simulink model "gait_testing"  (R2024a)
settings: Solver=ode23t  StartTime=0.0  StopTime=8  RelTol=1e-3  AbsTol=1e-3  EnableMultiTasking=on
model workspace (MAT data in the model file):
  A = 0.4
  Length_torso : Simulink.Parameter (value not decoded)
  Lower_limbs : Simulink.Parameter (value not decoded)
  Upper_limbs : Simulink.Parameter (value not decoded)
  Width_torso : Simulink.Parameter (value not decoded)
  f = 1.5
  r_foot : Simulink.Parameter (value not decoded)
  t_leg : Simulink.Parameter (value not decoded)
symbols that are objects in the model workspace (value not decoded): Length_torso, Lower_limbs, t_leg, Upper_limbs, Width_torso
undefined symbols (not defined in the file): P0x, P0z, P1x, P1z, P2x, P2z, X, Y, Z
libraries: sm_lib x88, functionAngles x16, functionAnglesSide x16, nesl_utility x15
(part 8 of 10)

== system gait_testing/Gait Selector/Trot Gait - Drive Function/left Front Hip gait/If Action Subsystem1 ==
  In1 : Inport
  tdur : Inport  Port=2
  Add : Sum  Inputs=+-
  Constant : Constant  Value=1.0 * pi
  Divide : Product  Inputs=*/
  Gain1 : Gain  Gain=2
  Gain4 : Gain  Gain=2*pi
  Sin : Trigonometry
  Out1 : Outport
  wires:
  Sin/1 -> Out1/1
  In1/1 -> Gain4/1
  Add/1 -> Gain1/1
  Constant/1 -> Add/2
  Gain1/1 -> Sin/1
  Gain4/1 -> Divide/1
  Divide/1 -> Add/1
  tdur/1 -> Divide/2

== system gait_testing/Gait Selector/Trot Gait - Drive Function/left Front Hip gait/If Action Subsystem2 ==
  In1 : Inport
  tdur : Inport  Port=2
  Add : Sum  Inputs=+-
  Constant : Constant  Value=1.25 * pi
  Divide : Product  Inputs=*/
  Gain1 : Gain  Gain=2/3
  Gain4 : Gain  Gain=2*pi
  Sin : Trigonometry  Operator=cos
  Out1 : Outport
  wires:
  Sin/1 -> Out1/1
  In1/1 -> Gain4/1
  Add/1 -> Gain1/1
  Constant/1 -> Add/2
  Gain1/1 -> Sin/1
  Gain4/1 -> Divide/1
  Divide/1 -> Add/1
  tdur/1 -> Divide/2

== system gait_testing/Gait Selector/Trot Gait - Drive Function/left Front Knee gait/If Action Subsystem4 ==
  In1 : Inport
  tdur : Inport  Port=2
  Add : Sum  Inputs=+-
  Constant : Constant  Value=0.75 * pi
  Divide : Product  Inputs=*/
  Gain1 : Gain  Gain=2
  Gain4 : Gain  Gain=2*pi
  Sin : Trigonometry
  Out1 : Outport
  wires:
  Sin/1 -> Out1/1
  In1/1 -> Gain4/1
  Add/1 -> Gain1/1
  Constant/1 -> Add/2
  Gain1/1 -> Sin/1
  Divide/1 -> Add/1
  Gain4/1 -> Divide/1
  tdur/1 -> Divide/2

== system gait_testing/Gait Selector/Trot Gait - Drive Function/right Back Hip gait/If Action Subsystem ==
  In1 : Inport
  tdur : Inport  Port=2
  Add : Sum  Inputs=+-
  Constant : Constant  Value=1.5 * pi
  Divide : Product  Inputs=*/
  Gain1 : Gain  Gain=2/3
  Gain4 : Gain  Gain=2*pi
  Sin : Trigonometry
  Out1 : Outport
  wires:
  In1/1 -> Gain4/1
  Constant/1 -> Add/2
  Add/1 -> Gain1/1
  Gain1/1 -> Sin/1
  Sin/1 -> Out1/1
  Gain4/1 -> Divide/1
  tdur/1 -> Divide/2
  Divide/1 -> Add/1

== system gait_testing/Gait Selector/Trot Gait - Drive Function/right Back Hip gait/If Action Subsystem1 ==
  In1 : Inport
  tdur : Inport  Port=2
  Add : Sum  Inputs=+-
  Constant : Constant  Value=1.0 * pi
  Divide : Product  Inputs=*/
  Gain1 : Gain  Gain=2
  Gain4 : Gain  Gain=2*pi
  Sin : Trigonometry
  Out1 : Outport
  wires:
  Sin/1 -> Out1/1
  In1/1 -> Gain4/1
  Add/1 -> Gain1/1
  Constant/1 -> Add/2
  Gain1/1 -> Sin/1
  Gain4/1 -> Divide/1
  Divide/1 -> Add/1
  tdur/1 -> Divide/2

== system gait_testing/Gait Selector/Trot Gait - Drive Function/right Back Hip gait/If Action Subsystem2 ==
  In1 : Inport
  tdur : Inport  Port=2
  Add : Sum  Inputs=+-
  Constant : Constant  Value=1.25 * pi
  Divide : Product  Inputs=*/
  Gain1 : Gain  Gain=2/3
  Gain4 : Gain  Gain=2*pi
  Sin : Trigonometry  Operator=cos
  Out1 : Outport
  wires:
  Sin/1 -> Out1/1
  In1/1 -> Gain4/1
  Add/1 -> Gain1/1
  Constant/1 -> Add/2
  Gain1/1 -> Sin/1
  Gain4/1 -> Divide/1
  Divide/1 -> Add/1
  tdur/1 -> Divide/2

== system gait_testing/Gait Selector/Trot Gait - Drive Function/right Back Knee gait/If Action Subsystem4 ==
  In1 : Inport
  tdur : Inport  Port=2
  Add : Sum  Inputs=+-
  Constant : Constant  Value=0.75 * pi
  Divide : Product  Inputs=*/
  Gain1 : Gain  Gain=2
  Gain4 : Gain  Gain=2*pi
  Sin : Trigonometry
  Out1 : Outport
  wires:
  Sin/1 -> Out1/1
  In1/1 -> Gain4/1
  Add/1 -> Gain1/1
  Constant/1 -> Add/2
  Gain1/1 -> Sin/1
  Divide/1 -> Add/1
  Gain4/1 -> Divide/1
  tdur/1 -> Divide/2

== system gait_testing/Gait Selector/Trot Gait - Drive Function/right Front Hip gait/If Action Subsystem ==
  In1 : Inport
  tdur : Inport  Port=2
  Add : Sum  Inputs=+-
  Constant : Constant  Value=1.5 * pi
  Divide : Product  Inputs=*/
  Gain1 : Gain  Gain=2/3
  Gain4 : Gain  Gain=2*pi
  Sin : Trigonometry
  Out1 : Outport
  wires:
  In1/1 -> Gain4/1
  Constant/1 -> Add/2
  Add/1 -> Gain1/1
  Gain1/1 -> Sin/1
  Sin/1 -> Out1/1
  Gain4/1 -> Divide/1
  tdur/1 -> Divide/2
  Divide/1 -> Add/1

== system gait_testing/Gait Selector/Trot Gait - Drive Function/right Front Hip gait/If Action Subsystem1 ==
  In1 : Inport
  tdur : Inport  Port=2
  Add : Sum  Inputs=+-
  Constant : Constant  Value=1.0 * pi
  Divide : Product  Inputs=*/
  Gain1 : Gain  Gain=2
  Gain4 : Gain  Gain=2*pi
  Sin : Trigonometry
  Out1 : Outport
  wires:
  Sin/1 -> Out1/1
  In1/1 -> Gain4/1
  Add/1 -> Gain1/1
  Constant/1 -> Add/2
  Gain1/1 -> Sin/1
  Gain4/1 -> Divide/1
  Divide/1 -> Add/1
  tdur/1 -> Divide/2

== system gait_testing/Gait Selector/Trot Gait - Drive Function/right Front Hip gait/If Action Subsystem2 ==
  In1 : Inport
  tdur : Inport  Port=2
  Add : Sum  Inputs=+-
  Constant : Constant  Value=1.25 * pi
  Divide : Product  Inputs=*/
  Gain1 : Gain  Gain=2/3
  Gain4 : Gain  Gain=2*pi
  Sin : Trigonometry  Operator=cos
  Out1 : Outport
  wires:
  Sin/1 -> Out1/1
  In1/1 -> Gain4/1
  Add/1 -> Gain1/1
  Constant/1 -> Add/2
  Gain1/1 -> Sin/1
  Gain4/1 -> Divide/1
  Divide/1 -> Add/1
  tdur/1 -> Divide/2

== system gait_testing/Gait Selector/Trot Gait - Drive Function/right Front Knee gait/If Action Subsystem4 ==
  In1 : Inport
  tdur : Inport  Port=2
  Add : Sum  Inputs=+-
  Constant : Constant  Value=0.75 * pi
  Divide : Product  Inputs=*/
  Gain1 : Gain  Gain=2
  Gain4 : Gain  Gain=2*pi
  Sin : Trigonometry
  Out1 : Outport
  wires:
  Sin/1 -> Out1/1
  In1/1 -> Gain4/1
  Add/1 -> Gain1/1
  Constant/1 -> Add/2
  Gain1/1 -> Sin/1
  Divide/1 -> Add/1
  Gain4/1 -> Divide/1
  tdur/1 -> Divide/2

== system gait_testing/Gait Selector/Turn Left Gait - Bezier Curves/Plane Movement/Subsystem1 ==
  X(t) : Inport
  Y(t) : Inport  Port=2
  Add : Sum  Inputs=+--+
  Add1 : Sum
  Add2 : Sum
  Asin : Trigonometry  Operator=asin
  Asin1 : Trigonometry  Operator=asin
  Cos : Trigonometry  Operator=acos
  Divide : Product  Inputs=*/
  Divide1 : Product  Inputs=*/
  Gain : Gain  Gain=1/(2*Upper_limbs*Lower_limbs)
  Gain1 : Gain  Gain=Lower_limbs
  Length lower Limb : Constant  Value=Lower_limbs
  Length upper Limb : Constant  Value=Upper_limbs
  Sin : Trigonometry
  Square{,1..3} (4 alike) : Math  Operator=square
  Square Root : Sqrt
  Theta1(X,Y) : Outport
  Theta2(X,Y) : Outport  Port=2
  wires:
  X(t)/1 -> Divide/1, Square/1
  Y(t)/1 -> Square1/1
  Square/1 -> Add1/1, Add/1
  Length upper Limb/1 -> Square2/1
  Length lower Limb/1 -> Square3/1
  Square2/1 -> Add/2
  Square3/1 -> Add/3
  Square1/1 -> Add1/2, Add/4
  Add/1 -> Gain/1
  Gain/1 -> Cos/1
  Cos/1 -> Theta2(X,Y)/1, Sin/1
  Asin/1 -> Add2/1
  Sin/1 -> Gain1/1
  Add1/1 -> Square Root/1
  Gain1/1 -> Divide1/1
  Square Root/1 -> Divide/2, Divide1/2
  Divide1/1 -> Asin1/1
  Asin1/1 -> Add2/2
  Add2/1 -> Theta1(X,Y)/1
  Divide/1 -> Asin/1

== system gait_testing/Gait Selector/Turn Left Gait - Bezier Curves/Plane Movement1/Subsystem1 ==
  X(t) : Inport
  Y(t) : Inport  Port=2
  Add : Sum  Inputs=+--+
  Add1 : Sum
  Add2 : Sum
  Asin : Trigonometry  Operator=asin
  Asin1 : Trigonometry  Operator=asin
  Cos : Trigonometry  Operator=acos
  Divide : Product  Inputs=*/
  Divide1 : Product  Inputs=*/
  Gain : Gain  Gain=1/(2*Upper_limbs*Lower_limbs)
  Gain1 : Gain  Gain=Lower_limbs
  Length lower Limb : Constant  Value=Lower_limbs
  Length upper Limb : Constant  Value=Upper_limbs
  Sin : Trigonometry
  Square{,1..3} (4 alike) : Math  Operator=square
  Square Root : Sqrt
  Theta1(X,Y) : Outport
  Theta2(X,Y) : Outport  Port=2
  wires:
  X(t)/1 -> Divide/1, Square/1
  Y(t)/1 -> Square1/1
  Square/1 -> Add1/1, Add/1
  Length upper Limb/1 -> Square2/1
  Length lower Limb/1 -> Square3/1
  Square2/1 -> Add/2
  Square3/1 -> Add/3
  Square1/1 -> Add1/2, Add/4
  Add/1 -> Gain/1
  Gain/1 -> Cos/1
  Cos/1 -> Theta2(X,Y)/1, Sin/1
  Asin/1 -> Add2/1
  Sin/1 -> Gain1/1
  Add1/1 -> Square Root/1
  Gain1/1 -> Divide1/1
  Square Root/1 -> Divide/2, Divide1/2
  Divide1/1 -> Asin1/1
  Asin1/1 -> Add2/2
  Add2/1 -> Theta1(X,Y)/1
  Divide/1 -> Asin/1

== system gait_testing/Gait Selector/Turn Left Gait - Bezier Curves/Plane Movement2/Subsystem1 ==
  X(t) : Inport
  Y(t) : Inport  Port=2
  Add : Sum  Inputs=+--+
  Add1 : Sum
  Add2 : Sum
  Asin : Trigonometry  Operator=asin
  Asin1 : Trigonometry  Operator=asin
  Cos : Trigonometry  Operator=acos
  Divide : Product  Inputs=*/
  Divide1 : Product  Inputs=*/
  Gain : Gain  Gain=1/(2*Upper_limbs*Lower_limbs)
  Gain1 : Gain  Gain=Lower_limbs
  Length lower Limb : Constant  Value=Lower_limbs
  Length upper Limb : Constant  Value=Upper_limbs
  Sin : Trigonometry
  Square{,1..3} (4 alike) : Math  Operator=square
  Square Root : Sqrt
  Theta1(X,Y) : Outport
  Theta2(X,Y) : Outport  Port=2
  wires:
  Divide/1 -> Asin/1
  Add2/1 -> Theta1(X,Y)/1
  Asin1/1 -> Add2/2
  Divide1/1 -> Asin1/1
  Square Root/1 -> Divide1/2, Divide/2
  Gain1/1 -> Divide1/1
  Add1/1 -> Square Root/1
  Sin/1 -> Gain1/1
  Asin/1 -> Add2/1
  Cos/1 -> Sin/1, Theta2(X,Y)/1
  Gain/1 -> Cos/1
  Add/1 -> Gain/1
  Square1/1 -> Add/4, Add1/2
  Square3/1 -> Add/3
  Square2/1 -> Add/2
  Length lower Limb/1 -> Square3/1
  Length upper Limb/1 -> Square2/1
  Square/1 -> Add/1, Add1/1
  Y(t)/1 -> Square1/1
  X(t)/1 -> Square/1, Divide/1

== system gait_testing/Gait Selector/Turn Left Gait - Bezier Curves/Plane Movement3/Subsystem1 ==
  X(t) : Inport
  Y(t) : Inport  Port=2
  Add : Sum  Inputs=+--+
  Add1 : Sum
  Add2 : Sum
  Asin : Trigonometry  Operator=asin
  Asin1 : Trigonometry  Operator=asin
  Cos : Trigonometry  Operator=acos
  Divide : Product  Inputs=*/
  Divide1 : Product  Inputs=*/
  Gain : Gain  Gain=1/(2*Upper_limbs*Lower_limbs)
  Gain1 : Gain  Gain=Lower_limbs
  Length lower Limb : Constant  Value=Lower_limbs
  Length upper Limb : Constant  Value=Upper_limbs
  Sin : Trigonometry
  Square{,1..3} (4 alike) : Math  Operator=square
  Square Root : Sqrt
  Theta1(X,Y) : Outport
  Theta2(X,Y) : Outport  Port=2
  wires:
  X(t)/1 -> Divide/1, Square/1
  Y(t)/1 -> Square1/1
  Square/1 -> Add1/1, Add/1
  Length upper Limb/1 -> Square2/1
  Length lower Limb/1 -> Square3/1
  Square2/1 -> Add/2
  Square3/1 -> Add/3
  Square1/1 -> Add1/2, Add/4
  Add/1 -> Gain/1
  Gain/1 -> Cos/1
  Cos/1 -> Theta2(X,Y)/1, Sin/1
  Asin/1 -> Add2/1
  Sin/1 -> Gain1/1
  Add1/1 -> Square Root/1
  Gain1/1 -> Divide1/1
  Square Root/1 -> Divide/2, Divide1/2
  Divide1/1 -> Asin1/1
  Asin1/1 -> Add2/2
  Add2/1 -> Theta1(X,Y)/1
  Divide/1 -> Asin/1

== system gait_testing/Gait Selector/Turn Left Gait - Bezier Curves/Plane Movement4/Subsystem1 ==
  X(t) : Inport
  Y(t) : Inport  Port=2
  Add : Sum  Inputs=+--+
  Add1 : Sum
  Add2 : Sum
  Asin : Trigonometry  Operator=asin
  Asin1 : Trigonometry  Operator=asin
  Cos : Trigonometry  Operator=acos
  Divide : Product  Inputs=*/
  Divide1 : Product  Inputs=*/
  Gain : Gain  Gain=1/(2*Upper_limbs*Lower_limbs)
  Gain1 : Gain  Gain=Lower_limbs
  Length lower Limb : Constant  Value=Lower_limbs
  Length upper Limb : Constant  Value=Upper_limbs
  Sin : Trigonometry
  Square{,1..3} (4 alike) : Math  Operator=square
  Square Root : Sqrt
  Theta1(X,Y) : Outport
  Theta2(X,Y) : Outport  Port=2
  wires:
  Divide/1 -> Asin/1
  Add2/1 -> Theta1(X,Y)/1
  Asin1/1 -> Add2/2
  Divide1/1 -> Asin1/1
  Square Root/1 -> Divide1/2, Divide/2
  Gain1/1 -> Divide1/1
  Add1/1 -> Square Root/1
  Sin/1 -> Gain1/1
  Asin/1 -> Add2/1
  Cos/1 -> Sin/1, Theta2(X,Y)/1
  Gain/1 -> Cos/1
  Add/1 -> Gain/1
  Square1/1 -> Add/4, Add1/2
  Square3/1 -> Add/3
  Square2/1 -> Add/2
  Length lower Limb/1 -> Square3/1
  Length upper Limb/1 -> Square2/1
  Square/1 -> Add/1, Add1/1
  Y(t)/1 -> Square1/1
  X(t)/1 -> Square/1, Divide/1

== system gait_testing/Gait Selector/Turn Left Gait - Bezier Curves/Sin-Movement/Subsystem1 ==
  X(t) : Inport
  Y(t) : Inport  Port=2
  Add : Sum  Inputs=+--+
  Add1 : Sum
  Add2 : Sum
  Asin : Trigonometry  Operator=asin
  Asin1 : Trigonometry  Operator=asin
  Cos : Trigonometry  Operator=acos
  Divide : Product  Inputs=*/
  Divide1 : Product  Inputs=*/
  Gain : Gain  Gain=1/(2*Upper_limbs*Lower_limbs)
  Gain1 : Gain  Gain=Lower_limbs
  Length lower Limb : Constant  Value=Lower_limbs
  Length upper Limb : Constant  Value=Upper_limbs
  Sin : Trigonometry
  Square{,1..3} (4 alike) : Math  Operator=square
  Square Root : Sqrt
  Theta1(X,Y) : Outport
  Theta2(X,Y) : Outport  Port=2
  wires:
  X(t)/1 -> Divide/1, Square/1
  Y(t)/1 -> Square1/1
  Square/1 -> Add1/1, Add/1
  Length upper Limb/1 -> Square2/1
  Length lower Limb/1 -> Square3/1
  Square2/1 -> Add/2
  Square3/1 -> Add/3
  Square1/1 -> Add1/2, Add/4
  Add/1 -> Gain/1
  Gain/1 -> Cos/1
  Cos/1 -> Theta2(X,Y)/1, Sin/1
  Asin/1 -> Add2/1
  Sin/1 -> Gain1/1
  Add1/1 -> Square Root/1
  Gain1/1 -> Divide1/1
  Square Root/1 -> Divide/2, Divide1/2
  Divide1/1 -> Asin1/1
  Asin1/1 -> Add2/2
  Add2/1 -> Theta1(X,Y)/1
  Divide/1 -> Asin/1

== system gait_testing/Gait Selector/Turn Left Gait - Bezier Curves/Stop when change/Triggered Subsystem ==
  t : Inport
  Action Port : ActionPort  InitializeStates=reset  ActionPortLabel=case [ 1 ]:
  MATLAB Function : MATLAB Function  TreatAsAtomicUnit=on
  Change Time : Outport
  wires:
  MATLAB Function/1(activationTime) -> Change Time/1
  t/1 -> MATLAB Function/1(u)

== system gait_testing/Gait Selector/Turn Left Gait - Bezier Curves/delay and stop when change/Triggered Subsystem ==
  t : Inport
  Action Port : ActionPort  InitializeStates=reset  ActionPortLabel=case [ 1 ]:
  MATLAB Function : MATLAB Function  TreatAsAtomicUnit=on
  Change Time : Outport
  wires:
  MATLAB Function/1(activationTime) -> Change Time/1
  t/1 -> MATLAB Function/1(u)

== system gait_testing/Gait Selector/Turn Left Gait - Bezier Curves/delay and stop when change1/Triggered Subsystem ==
  t : Inport
  Action Port : ActionPort  InitializeStates=reset  ActionPortLabel=case [ 1 ]:
  MATLAB Function : MATLAB Function  TreatAsAtomicUnit=on
  Change Time : Outport
  wires:
  MATLAB Function/1(activationTime) -> Change Time/1
  t/1 -> MATLAB Function/1(u)

== system gait_testing/Gait Selector/Turn Left Gait - Bezier Curves/delay and stop when change2/Triggered Subsystem ==
  t : Inport
  Action Port : ActionPort  InitializeStates=reset  ActionPortLabel=case [ 1 ]:
  MATLAB Function : MATLAB Function  TreatAsAtomicUnit=on
  Change Time : Outport
  wires:
  MATLAB Function/1(activationTime) -> Change Time/1
  t/1 -> MATLAB Function/1(u)

== system gait_testing/Gait Selector/Turn Right Gait - Bezier Curves/Plane Movement/Subsystem1 ==
  X(t) : Inport
  Y(t) : Inport  Port=2
  Add : Sum  Inputs=+--+
  Add1 : Sum
  Add2 : Sum
  Asin : Trigonometry  Operator=asin
  Asin1 : Trigonometry  Operator=asin
  Cos : Trigonometry  Operator=acos
  Divide : Product  Inputs=*/
  Divide1 : Product  Inputs=*/
  Gain : Gain  Gain=1/(2*Upper_limbs*Lower_limbs)
  Gain1 : Gain  Gain=Lower_limbs
  Length lower Limb : Constant  Value=Lower_limbs
  Length upper Limb : Constant  Value=Upper_limbs
  Sin : Trigonometry
  Square{,1..3} (4 alike) : Math  Operator=square
  Square Root : Sqrt
  Theta1(X,Y) : Outport
  Theta2(X,Y) : Outport  Port=2
  wires:
  Divide/1 -> Asin/1
  Add2/1 -> Theta1(X,Y)/1
  Asin1/1 -> Add2/2
  Divide1/1 -> Asin1/1
  Square Root/1 -> Divide1/2, Divide/2
  Gain1/1 -> Divide1/1
  Add1/1 -> Square Root/1
  Sin/1 -> Gain1/1
  Asin/1 -> Add2/1
  Cos/1 -> Sin/1, Theta2(X,Y)/1
  Gain/1 -> Cos/1
  Add/1 -> Gain/1
  Square1/1 -> Add/4, Add1/2
  Square3/1 -> Add/3
  Square2/1 -> Add/2
  Length lower Limb/1 -> Square3/1
  Length upper Limb/1 -> Square2/1
  Square/1 -> Add/1, Add1/1
  Y(t)/1 -> Square1/1
  X(t)/1 -> Square/1, Divide/1

== system gait_testing/Gait Selector/Turn Right Gait - Bezier Curves/Plane Movement1/Subsystem1 ==
  X(t) : Inport
  Y(t) : Inport  Port=2
  Add : Sum  Inputs=+--+
  Add1 : Sum
  Add2 : Sum
  Asin : Trigonometry  Operator=asin
  Asin1 : Trigonometry  Operator=asin
  Cos : Trigonometry  Operator=acos
  Divide : Product  Inputs=*/
  Divide1 : Product  Inputs=*/
  Gain : Gain  Gain=1/(2*Upper_limbs*Lower_limbs)
  Gain1 : Gain  Gain=Lower_limbs
  Length lower Limb : Constant  Value=Lower_limbs
  Length upper Limb : Constant  Value=Upper_limbs
  Sin : Trigonometry
  Square{,1..3} (4 alike) : Math  Operator=square
  Square Root : Sqrt
  Theta1(X,Y) : Outport
  Theta2(X,Y) : Outport  Port=2
  wires:
  Divide/1 -> Asin/1
  Add2/1 -> Theta1(X,Y)/1
  Asin1/1 -> Add2/2
  Divide1/1 -> Asin1/1
  Square Root/1 -> Divide1/2, Divide/2
  Gain1/1 -> Divide1/1
  Add1/1 -> Square Root/1
  Sin/1 -> Gain1/1
  Asin/1 -> Add2/1
  Cos/1 -> Sin/1, Theta2(X,Y)/1
  Gain/1 -> Cos/1
  Add/1 -> Gain/1
  Square1/1 -> Add/4, Add1/2
  Square3/1 -> Add/3
  Square2/1 -> Add/2
  Length lower Limb/1 -> Square3/1
  Length upper Limb/1 -> Square2/1
  Square/1 -> Add/1, Add1/1
  Y(t)/1 -> Square1/1
  X(t)/1 -> Square/1, Divide/1

== system gait_testing/Gait Selector/Turn Right Gait - Bezier Curves/Plane Movement2/Subsystem1 ==
  X(t) : Inport
  Y(t) : Inport  Port=2
  Add : Sum  Inputs=+--+
  Add1 : Sum
  Add2 : Sum
  Asin : Trigonometry  Operator=asin
  Asin1 : Trigonometry  Operator=asin
  Cos : Trigonometry  Operator=acos
  Divide : Product  Inputs=*/
  Divide1 : Product  Inputs=*/
  Gain : Gain  Gain=1/(2*Upper_limbs*Lower_limbs)
  Gain1 : Gain  Gain=Lower_limbs
  Length lower Limb : Constant  Value=Lower_limbs
  Length upper Limb : Constant  Value=Upper_limbs
  Sin : Trigonometry
  Square{,1..3} (4 alike) : Math  Operator=square
  Square Root : Sqrt
  Theta1(X,Y) : Outport
  Theta2(X,Y) : Outport  Port=2
  wires:
  X(t)/1 -> Divide/1, Square/1
  Y(t)/1 -> Square1/1
  Square/1 -> Add1/1, Add/1
  Length upper Limb/1 -> Square2/1
  Length lower Limb/1 -> Square3/1
  Square2/1 -> Add/2
  Square3/1 -> Add/3
  Square1/1 -> Add1/2, Add/4
  Add/1 -> Gain/1
  Gain/1 -> Cos/1
  Cos/1 -> Theta2(X,Y)/1, Sin/1
  Asin/1 -> Add2/1
  Sin/1 -> Gain1/1
  Add1/1 -> Square Root/1
  Gain1/1 -> Divide1/1
  Square Root/1 -> Divide/2, Divide1/2
  Divide1/1 -> Asin1/1
  Asin1/1 -> Add2/2
  Add2/1 -> Theta1(X,Y)/1
  Divide/1 -> Asin/1

== system gait_testing/Gait Selector/Turn Right Gait - Bezier Curves/Plane Movement3/Subsystem1 ==
  X(t) : Inport
  Y(t) : Inport  Port=2
  Add : Sum  Inputs=+--+
  Add1 : Sum
  Add2 : Sum
  Asin : Trigonometry  Operator=asin
  Asin1 : Trigonometry  Operator=asin
  Cos : Trigonometry  Operator=acos
  Divide : Product  Inputs=*/
  Divide1 : Product  Inputs=*/
  Gain : Gain  Gain=1/(2*Upper_limbs*Lower_limbs)
  Gain1 : Gain  Gain=Lower_limbs
  Length lower Limb : Constant  Value=Lower_limbs
  Length upper Limb : Constant  Value=Upper_limbs
  Sin : Trigonometry
  Square{,1..3} (4 alike) : Math  Operator=square
  Square Root : Sqrt
  Theta1(X,Y) : Outport
  Theta2(X,Y) : Outport  Port=2
  wires:
  X(t)/1 -> Divide/1, Square/1
  Y(t)/1 -> Square1/1
  Square/1 -> Add1/1, Add/1
  Length upper Limb/1 -> Square2/1
  Length lower Limb/1 -> Square3/1
  Square2/1 -> Add/2
  Square3/1 -> Add/3
  Square1/1 -> Add1/2, Add/4
  Add/1 -> Gain/1
  Gain/1 -> Cos/1
  Cos/1 -> Theta2(X,Y)/1, Sin/1
  Asin/1 -> Add2/1
  Sin/1 -> Gain1/1
  Add1/1 -> Square Root/1
  Gain1/1 -> Divide1/1
  Square Root/1 -> Divide/2, Divide1/2
  Divide1/1 -> Asin1/1
  Asin1/1 -> Add2/2
  Add2/1 -> Theta1(X,Y)/1
  Divide/1 -> Asin/1

== system gait_testing/Gait Selector/Turn Right Gait - Bezier Curves/Plane Movement4/Subsystem1 ==
  X(t) : Inport
  Y(t) : Inport  Port=2
  Add : Sum  Inputs=+--+
  Add1 : Sum
  Add2 : Sum
  Asin : Trigonometry  Operator=asin
  Asin1 : Trigonometry  Operator=asin
  Cos : Trigonometry  Operator=acos
  Divide : Product  Inputs=*/
  Divide1 : Product  Inputs=*/
  Gain : Gain  Gain=1/(2*Upper_limbs*Lower_limbs)
  Gain1 : Gain  Gain=Lower_limbs
  Length lower Limb : Constant  Value=Lower_limbs
  Length upper Limb : Constant  Value=Upper_limbs
  Sin : Trigonometry
  Square{,1..3} (4 alike) : Math  Operator=square
  Square Root : Sqrt
  Theta1(X,Y) : Outport
  Theta2(X,Y) : Outport  Port=2
  wires:
  X(t)/1 -> Divide/1, Square/1
  Y(t)/1 -> Square1/1
  Square/1 -> Add1/1, Add/1
  Length upper Limb/1 -> Square2/1
  Length lower Limb/1 -> Square3/1
  Square2/1 -> Add/2
  Square3/1 -> Add/3
  Square1/1 -> Add1/2, Add/4
  Add/1 -> Gain/1
  Gain/1 -> Cos/1
  Cos/1 -> Theta2(X,Y)/1, Sin/1
  Asin/1 -> Add2/1
  Sin/1 -> Gain1/1
  Add1/1 -> Square Root/1
  Gain1/1 -> Divide1/1
  Square Root/1 -> Divide/2, Divide1/2
  Divide1/1 -> Asin1/1
  Asin1/1 -> Add2/2
  Add2/1 -> Theta1(X,Y)/1
  Divide/1 -> Asin/1

== system gait_testing/Gait Selector/Turn Right Gait - Bezier Curves/Sin-Movement/Subsystem1 ==
  X(t) : Inport
  Y(t) : Inport  Port=2
  Add : Sum  Inputs=+--+
  Add1 : Sum
  Add2 : Sum
  Asin : Trigonometry  Operator=asin
  Asin1 : Trigonometry  Operator=asin
  Cos : Trigonometry  Operator=acos
  Divide : Product  Inputs=*/
  Divide1 : Product  Inputs=*/
  Gain : Gain  Gain=1/(2*Upper_limbs*Lower_limbs)
  Gain1 : Gain  Gain=Lower_limbs
  Length lower Limb : Constant  Value=Lower_limbs
  Length upper Limb : Constant  Value=Upper_limbs
  Sin : Trigonometry
  Square{,1..3} (4 alike) : Math  Operator=square
  Square Root : Sqrt
  Theta1(X,Y) : Outport
  Theta2(X,Y) : Outport  Port=2
  wires:
  Divide/1 -> Asin/1
  Add2/1 -> Theta1(X,Y)/1
  Asin1/1 -> Add2/2
  Divide1/1 -> Asin1/1
  Square Root/1 -> Divide1/2, Divide/2
  Gain1/1 -> Divide1/1
  Add1/1 -> Square Root/1
  Sin/1 -> Gain1/1
  Asin/1 -> Add2/1
  Cos/1 -> Sin/1, Theta2(X,Y)/1
  Gain/1 -> Cos/1
  Add/1 -> Gain/1
  Square1/1 -> Add/4, Add1/2
  Square3/1 -> Add/3
  Square2/1 -> Add/2
  Length lower Limb/1 -> Square3/1
  Length upper Limb/1 -> Square2/1
  Square/1 -> Add/1, Add1/1
  Y(t)/1 -> Square1/1
  X(t)/1 -> Square/1, Divide/1

== system gait_testing/Gait Selector/Turn Right Gait - Bezier Curves/Stop when change/Triggered Subsystem ==
  t : Inport
  Action Port : ActionPort  InitializeStates=reset  ActionPortLabel=case [ 1 ]:
  MATLAB Function : MATLAB Function  TreatAsAtomicUnit=on
  Change Time : Outport
  wires:
  MATLAB Function/1(activationTime) -> Change Time/1
  t/1 -> MATLAB Function/1(u)

== system gait_testing/Gait Selector/Turn Right Gait - Bezier Curves/delay and stop when change/Triggered Subsystem ==
  t : Inport
  Action Port : ActionPort  InitializeStates=reset  ActionPortLabel=case [ 1 ]:
  MATLAB Function : MATLAB Function  TreatAsAtomicUnit=on
  Change Time : Outport
  wires:
  MATLAB Function/1(activationTime) -> Change Time/1
  t/1 -> MATLAB Function/1(u)

== system gait_testing/Gait Selector/Turn Right Gait - Bezier Curves/delay and stop when change1/Triggered Subsystem ==
  t : Inport
  Action Port : ActionPort  InitializeStates=reset  ActionPortLabel=case [ 1 ]:
  MATLAB Function : MATLAB Function  TreatAsAtomicUnit=on
  Change Time : Outport
  wires:
  MATLAB Function/1(activationTime) -> Change Time/1
  t/1 -> MATLAB Function/1(u)

== system gait_testing/Gait Selector/Turn Right Gait - Bezier Curves/delay and stop when change2/Triggered Subsystem ==
  t : Inport
  Action Port : ActionPort  InitializeStates=reset  ActionPortLabel=case [ 1 ]:
  MATLAB Function : MATLAB Function  TreatAsAtomicUnit=on
  Change Time : Outport
  wires:
  MATLAB Function/1(activationTime) -> Change Time/1
  t/1 -> MATLAB Function/1(u)

== system gait_testing/Gait Selector/Walk Back Gait - Bezier Curves/Plane Movement/Subsystem1 ==
  X(t) : Inport
  Y(t) : Inport  Port=2
  Add : Sum  Inputs=+--+
  Add1 : Sum
  Add2 : Sum
  Asin : Trigonometry  Operator=asin
  Asin1 : Trigonometry  Operator=asin
  Cos : Trigonometry  Operator=acos
  Divide : Product  Inputs=*/
  Divide1 : Product  Inputs=*/
  Gain : Gain  Gain=1/(2*Upper_limbs*Lower_limbs)
  Gain1 : Gain  Gain=Lower_limbs
  Length lower Limb : Constant  Value=Lower_limbs
  Length upper Limb : Constant  Value=Upper_limbs
  Sin : Trigonometry
  Square{,1..3} (4 alike) : Math  Operator=square
  Square Root : Sqrt
  Theta1(X,Y) : Outport
  Theta2(X,Y) : Outport  Port=2
  wires:
  Divide/1 -> Asin/1
  Add2/1 -> Theta1(X,Y)/1
  Asin1/1 -> Add2/2
  Divide1/1 -> Asin1/1
  Square Root/1 -> Divide1/2, Divide/2
  Gain1/1 -> Divide1/1
  Add1/1 -> Square Root/1
  Sin/1 -> Gain1/1
  Asin/1 -> Add2/1
  Cos/1 -> Sin/1, Theta2(X,Y)/1
  Gain/1 -> Cos/1
  Add/1 -> Gain/1
  Square1/1 -> Add/4, Add1/2
  Square3/1 -> Add/3
  Square2/1 -> Add/2
  Length lower Limb/1 -> Square3/1
  Length upper Limb/1 -> Square2/1
  Square/1 -> Add/1, Add1/1
  Y(t)/1 -> Square1/1
  X(t)/1 -> Square/1, Divide/1

== system gait_testing/Gait Selector/Walk Back Gait - Bezier Curves/Plane Movement1/Subsystem1 ==
  X(t) : Inport
  Y(t) : Inport  Port=2
  Add : Sum  Inputs=+--+
  Add1 : Sum
  Add2 : Sum
  Asin : Trigonometry  Operator=asin
  Asin1 : Trigonometry  Operator=asin
  Cos : Trigonometry  Operator=acos
  Divide : Product  Inputs=*/
  Divide1 : Product  Inputs=*/
  Gain : Gain  Gain=1/(2*Upper_limbs*Lower_limbs)
  Gain1 : Gain  Gain=Lower_limbs
  Length lower Limb : Constant  Value=Lower_limbs
  Length upper Limb : Constant  Value=Upper_limbs
  Sin : Trigonometry
  Square{,1..3} (4 alike) : Math  Operator=square
  Square Root : Sqrt
  Theta1(X,Y) : Outport
  Theta2(X,Y) : Outport  Port=2
  wires:
  Divide/1 -> Asin/1
  Add2/1 -> Theta1(X,Y)/1
  Asin1/1 -> Add2/2
  Divide1/1 -> Asin1/1
  Square Root/1 -> Divide1/2, Divide/2
  Gain1/1 -> Divide1/1
  Add1/1 -> Square Root/1
  Sin/1 -> Gain1/1
  Asin/1 -> Add2/1
  Cos/1 -> Sin/1, Theta2(X,Y)/1
  Gain/1 -> Cos/1
  Add/1 -> Gain/1
  Square1/1 -> Add/4, Add1/2
  Square3/1 -> Add/3
  Square2/1 -> Add/2
  Length lower Limb/1 -> Square3/1
  Length upper Limb/1 -> Square2/1
  Square/1 -> Add/1, Add1/1
  Y(t)/1 -> Square1/1
  X(t)/1 -> Square/1, Divide/1

== system gait_testing/Gait Selector/Walk Back Gait - Bezier Curves/Plane Movement2/Subsystem1 ==
  X(t) : Inport
  Y(t) : Inport  Port=2
  Add : Sum  Inputs=+--+
  Add1 : Sum
  Add2 : Sum
  Asin : Trigonometry  Operator=asin
  Asin1 : Trigonometry  Operator=asin
  Cos : Trigonometry  Operator=acos
  Divide : Product  Inputs=*/
  Divide1 : Product  Inputs=*/
  Gain : Gain  Gain=1/(2*Upper_limbs*Lower_limbs)
  Gain1 : Gain  Gain=Lower_limbs
  Length lower Limb : Constant  Value=Lower_limbs
  Length upper Limb : Constant  Value=Upper_limbs
  Sin : Trigonometry
  Square{,1..3} (4 alike) : Math  Operator=square
  Square Root : Sqrt
  Theta1(X,Y) : Outport
  Theta2(X,Y) : Outport  Port=2
  wires:
  X(t)/1 -> Divide/1, Square/1
  Y(t)/1 -> Square1/1
  Square/1 -> Add1/1, Add/1
  Length upper Limb/1 -> Square2/1
  Length lower Limb/1 -> Square3/1
  Square2/1 -> Add/2
  Square3/1 -> Add/3
  Square1/1 -> Add1/2, Add/4
  Add/1 -> Gain/1
  Gain/1 -> Cos/1
  Cos/1 -> Theta2(X,Y)/1, Sin/1
  Asin/1 -> Add2/1
  Sin/1 -> Gain1/1
  Add1/1 -> Square Root/1
  Gain1/1 -> Divide1/1
  Square Root/1 -> Divide/2, Divide1/2
  Divide1/1 -> Asin1/1
  Asin1/1 -> Add2/2
  Add2/1 -> Theta1(X,Y)/1
  Divide/1 -> Asin/1

== system gait_testing/Gait Selector/Walk Back Gait - Bezier Curves/Plane Movement3/Subsystem1 ==
  X(t) : Inport
  Y(t) : Inport  Port=2
  Add : Sum  Inputs=+--+
  Add1 : Sum
  Add2 : Sum
  Asin : Trigonometry  Operator=asin
  Asin1 : Trigonometry  Operator=asin
  Cos : Trigonometry  Operator=acos
  Divide : Product  Inputs=*/
  Divide1 : Product  Inputs=*/
  Gain : Gain  Gain=1/(2*Upper_limbs*Lower_limbs)
  Gain1 : Gain  Gain=Lower_limbs
  Length lower Limb : Constant  Value=Lower_limbs
  Length upper Limb : Constant  Value=Upper_limbs
  Sin : Trigonometry
  Square{,1..3} (4 alike) : Math  Operator=square
  Square Root : Sqrt
  Theta1(X,Y) : Outport
  Theta2(X,Y) : Outport  Port=2
  wires:
  Divide/1 -> Asin/1
  Add2/1 -> Theta1(X,Y)/1
  Asin1/1 -> Add2/2
  Divide1/1 -> Asin1/1
  Square Root/1 -> Divide1/2, Divide/2
  Gain1/1 -> Divide1/1
  Add1/1 -> Square Root/1
  Sin/1 -> Gain1/1
  Asin/1 -> Add2/1
  Cos/1 -> Sin/1, Theta2(X,Y)/1
  Gain/1 -> Cos/1
  Add/1 -> Gain/1
  Square1/1 -> Add/4, Add1/2
  Square3/1 -> Add/3
  Square2/1 -> Add/2
  Length lower Limb/1 -> Square3/1
  Length upper Limb/1 -> Square2/1
  Square/1 -> Add/1, Add1/1
  Y(t)/1 -> Square1/1
  X(t)/1 -> Square/1, Divide/1

== system gait_testing/Gait Selector/Walk Back Gait - Bezier Curves/Plane Movement4/Subsystem1 ==
  X(t) : Inport
  Y(t) : Inport  Port=2
  Add : Sum  Inputs=+--+
  Add1 : Sum
  Add2 : Sum
  Asin : Trigonometry  Operator=asin
  Asin1 : Trigonometry  Operator=asin
  Cos : Trigonometry  Operator=acos
  Divide : Product  Inputs=*/
  Divide1 : Product  Inputs=*/
  Gain : Gain  Gain=1/(2*Upper_limbs*Lower_limbs)
  Gain1 : Gain  Gain=Lower_limbs
  Length lower Limb : Constant  Value=Lower_limbs
  Length upper Limb : Constant  Value=Upper_limbs
  Sin : Trigonometry
  Square{,1..3} (4 alike) : Math  Operator=square
  Square Root : Sqrt
  Theta1(X,Y) : Outport
  Theta2(X,Y) : Outport  Port=2
  wires:
  X(t)/1 -> Divide/1, Square/1
  Y(t)/1 -> Square1/1
  Square/1 -> Add1/1, Add/1
  Length upper Limb/1 -> Square2/1
  Length lower Limb/1 -> Square3/1
  Square2/1 -> Add/2
  Square3/1 -> Add/3
  Square1/1 -> Add1/2, Add/4
  Add/1 -> Gain/1
  Gain/1 -> Cos/1
  Cos/1 -> Theta2(X,Y)/1, Sin/1
  Asin/1 -> Add2/1
  Sin/1 -> Gain1/1
  Add1/1 -> Square Root/1
  Gain1/1 -> Divide1/1
  Square Root/1 -> Divide/2, Divide1/2
  Divide1/1 -> Asin1/1
  Asin1/1 -> Add2/2
  Add2/1 -> Theta1(X,Y)/1
  Divide/1 -> Asin/1

== system gait_testing/Gait Selector/Walk Back Gait - Bezier Curves/Sin-Movement/Subsystem1 ==
  X(t) : Inport
  Y(t) : Inport  Port=2
  Add : Sum  Inputs=+--+
  Add1 : Sum
  Add2 : Sum
  Asin : Trigonometry  Operator=asin
  Asin1 : Trigonometry  Operator=asin
  Cos : Trigonometry  Operator=acos
  Divide : Product  Inputs=*/
  Divide1 : Product  Inputs=*/
  Gain : Gain  Gain=1/(2*Upper_limbs*Lower_limbs)
  Gain1 : Gain  Gain=Lower_limbs
  Length lower Limb : Constant  Value=Lower_limbs
  Length upper Limb : Constant  Value=Upper_limbs
  Sin : Trigonometry
  Square{,1..3} (4 alike) : Math  Operator=square
  Square Root : Sqrt
  Theta1(X,Y) : Outport
  Theta2(X,Y) : Outport  Port=2
  wires:
  Divide/1 -> Asin/1
  Add2/1 -> Theta1(X,Y)/1
  Asin1/1 -> Add2/2
  Divide1/1 -> Asin1/1
  Square Root/1 -> Divide1/2, Divide/2
  Gain1/1 -> Divide1/1
  Add1/1 -> Square Root/1
  Sin/1 -> Gain1/1
  Asin/1 -> Add2/1
  Cos/1 -> Sin/1, Theta2(X,Y)/1
  Gain/1 -> Cos/1
  Add/1 -> Gain/1
  Square1/1 -> Add/4, Add1/2
  Square3/1 -> Add/3
  Square2/1 -> Add/2
  Length lower Limb/1 -> Square3/1
  Length upper Limb/1 -> Square2/1
  Square/1 -> Add/1, Add1/1
  Y(t)/1 -> Square1/1
  X(t)/1 -> Square/1, Divide/1

== system gait_testing/Gait Selector/Walk Back Gait - Bezier Curves/Stop when change/Triggered Subsystem ==
  t : Inport
  Action Port : ActionPort  InitializeStates=reset  ActionPortLabel=case [ 1 ]:
  MATLAB Function : MATLAB Function  TreatAsAtomicUnit=on
  Change Time : Outport
  wires:
  MATLAB Function/1(activationTime) -> Change Time/1
  t/1 -> MATLAB Function/1(u)

== system gait_testing/Gait Selector/Walk Back Gait - Bezier Curves/delay and stop when change/Triggered Subsystem ==
  t : Inport
  Action Port : ActionPort  InitializeStates=reset  ActionPortLabel=case [ 1 ]:
  MATLAB Function : MATLAB Function  TreatAsAtomicUnit=on
  Change Time : Outport
  wires:
  MATLAB Function/1(activationTime) -> Change Time/1
  t/1 -> MATLAB Function/1(u)

== system gait_testing/Gait Selector/Walk Back Gait - Bezier Curves/delay and stop when change1/Triggered Subsystem ==
  t : Inport
  Action Port : ActionPort  InitializeStates=reset  ActionPortLabel=case [ 1 ]:
  MATLAB Function : MATLAB Function  TreatAsAtomicUnit=on
  Change Time : Outport
  wires:
  MATLAB Function/1(activationTime) -> Change Time/1
  t/1 -> MATLAB Function/1(u)

== system gait_testing/Gait Selector/Walk Back Gait - Bezier Curves/delay and stop when change2/Triggered Subsystem ==
  t : Inport
  Action Port : ActionPort  InitializeStates=reset  ActionPortLabel=case [ 1 ]:
  MATLAB Function : MATLAB Function  TreatAsAtomicUnit=on
  Change Time : Outport
  wires:
  MATLAB Function/1(activationTime) -> Change Time/1
  t/1 -> MATLAB Function/1(u)

== system gait_testing/Gait Selector/Walk Gait - Bezier Curves/Plane Movement/Subsystem1 ==
  X(t) : Inport
  Y(t) : Inport  Port=2
  Add : Sum  Inputs=+--+
  Add1 : Sum
  Add2 : Sum
  Asin : Trigonometry  Operator=asin
  Asin1 : Trigonometry  Operator=asin
  Cos : Trigonometry  Operator=acos
  Divide : Product  Inputs=*/
  Divide1 : Product  Inputs=*/
  Gain : Gain  Gain=1/(2*Upper_limbs*Lower_limbs)
  Gain1 : Gain  Gain=Lower_limbs
  Length lower Limb : Constant  Value=Lower_limbs
  Length upper Limb : Constant  Value=Upper_limbs
  Sin : Trigonometry
  Square{,1..3} (4 alike) : Math  Operator=square
  Square Root : Sqrt
  Theta1(X,Y) : Outport
  Theta2(X,Y) : Outport  Port=2
  wires:
  Divide/1 -> Asin/1
  Add2/1 -> Theta1(X,Y)/1
  Asin1/1 -> Add2/2
  Divide1/1 -> Asin1/1
  Square Root/1 -> Divide1/2, Divide/2
  Gain1/1 -> Divide1/1
  Add1/1 -> Square Root/1
  Sin/1 -> Gain1/1
  Asin/1 -> Add2/1
  Cos/1 -> Sin/1, Theta2(X,Y)/1
  Gain/1 -> Cos/1
  Add/1 -> Gain/1
  Square1/1 -> Add/4, Add1/2
  Square3/1 -> Add/3
  Square2/1 -> Add/2
  Length lower Limb/1 -> Square3/1
  Length upper Limb/1 -> Square2/1
  Square/1 -> Add/1, Add1/1
  Y(t)/1 -> Square1/1
  X(t)/1 -> Square/1, Divide/1

== system gait_testing/Gait Selector/Walk Gait - Bezier Curves/Plane Movement1/Subsystem1 ==
  X(t) : Inport
  Y(t) : Inport  Port=2
  Add : Sum  Inputs=+--+
  Add1 : Sum
  Add2 : Sum
  Asin : Trigonometry  Operator=asin
  Asin1 : Trigonometry  Operator=asin
  Cos : Trigonometry  Operator=acos
  Divide : Product  Inputs=*/
  Divide1 : Product  Inputs=*/
  Gain : Gain  Gain=1/(2*Upper_limbs*Lower_limbs)
  Gain1 : Gain  Gain=Lower_limbs
  Length lower Limb : Constant  Value=Lower_limbs
  Length upper Limb : Constant  Value=Upper_limbs
  Sin : Trigonometry
  Square{,1..3} (4 alike) : Math  Operator=square
  Square Root : Sqrt
  Theta1(X,Y) : Outport
  Theta2(X,Y) : Outport  Port=2
  wires:
  X(t)/1 -> Divide/1, Square/1
  Y(t)/1 -> Square1/1
  Square/1 -> Add1/1, Add/1
  Length upper Limb/1 -> Square2/1
  Length lower Limb/1 -> Square3/1
  Square2/1 -> Add/2
  Square3/1 -> Add/3
  Square1/1 -> Add1/2, Add/4
  Add/1 -> Gain/1
  Gain/1 -> Cos/1
  Cos/1 -> Theta2(X,Y)/1, Sin/1
  Asin/1 -> Add2/1
  Sin/1 -> Gain1/1
  Add1/1 -> Square Root/1
  Gain1/1 -> Divide1/1
  Square Root/1 -> Divide/2, Divide1/2
  Divide1/1 -> Asin1/1
  Asin1/1 -> Add2/2
  Add2/1 -> Theta1(X,Y)/1
  Divide/1 -> Asin/1

== system gait_testing/Gait Selector/Walk Gait - Bezier Curves/Plane Movement2/Subsystem1 ==
  X(t) : Inport
  Y(t) : Inport  Port=2
  Add : Sum  Inputs=+--+
  Add1 : Sum
  Add2 : Sum
  Asin : Trigonometry  Operator=asin
  Asin1 : Trigonometry  Operator=asin
  Cos : Trigonometry  Operator=acos
  Divide : Product  Inputs=*/
  Divide1 : Product  Inputs=*/
  Gain : Gain  Gain=1/(2*Upper_limbs*Lower_limbs)
  Gain1 : Gain  Gain=Lower_limbs
  Length lower Limb : Constant  Value=Lower_limbs
  Length upper Limb : Constant  Value=Upper_limbs
  Sin : Trigonometry
  Square{,1..3} (4 alike) : Math  Operator=square
  Square Root : Sqrt
  Theta1(X,Y) : Outport
  Theta2(X,Y) : Outport  Port=2
  wires:
  X(t)/1 -> Divide/1, Square/1
  Y(t)/1 -> Square1/1
  Square/1 -> Add1/1, Add/1
  Length upper Limb/1 -> Square2/1
  Length lower Limb/1 -> Square3/1
  Square2/1 -> Add/2
  Square3/1 -> Add/3
  Square1/1 -> Add1/2, Add/4
  Add/1 -> Gain/1
  Gain/1 -> Cos/1
  Cos/1 -> Theta2(X,Y)/1, Sin/1
  Asin/1 -> Add2/1
  Sin/1 -> Gain1/1
  Add1/1 -> Square Root/1
  Gain1/1 -> Divide1/1
  Square Root/1 -> Divide/2, Divide1/2
  Divide1/1 -> Asin1/1
  Asin1/1 -> Add2/2
  Add2/1 -> Theta1(X,Y)/1
  Divide/1 -> Asin/1

== system gait_testing/Gait Selector/Walk Gait - Bezier Curves/Plane Movement3/Subsystem1 ==
  X(t) : Inport
  Y(t) : Inport  Port=2
  Add : Sum  Inputs=+--+
  Add1 : Sum
  Add2 : Sum
  Asin : Trigonometry  Operator=asin
  Asin1 : Trigonometry  Operator=asin
  Cos : Trigonometry  Operator=acos
  Divide : Product  Inputs=*/
  Divide1 : Product  Inputs=*/
  Gain : Gain  Gain=1/(2*Upper_limbs*Lower_limbs)
  Gain1 : Gain  Gain=Lower_limbs
  Length lower Limb : Constant  Value=Lower_limbs
  Length upper Limb : Constant  Value=Upper_limbs
  Sin : Trigonometry
  Square{,1..3} (4 alike) : Math  Operator=square
  Square Root : Sqrt
  Theta1(X,Y) : Outport
  Theta2(X,Y) : Outport  Port=2
  wires:
  Divide/1 -> Asin/1
  Add2/1 -> Theta1(X,Y)/1
  Asin1/1 -> Add2/2
  Divide1/1 -> Asin1/1
  Square Root/1 -> Divide1/2, Divide/2
  Gain1/1 -> Divide1/1
  Add1/1 -> Square Root/1
  Sin/1 -> Gain1/1
  Asin/1 -> Add2/1
  Cos/1 -> Sin/1, Theta2(X,Y)/1
  Gain/1 -> Cos/1
  Add/1 -> Gain/1
  Square1/1 -> Add/4, Add1/2
  Square3/1 -> Add/3
  Square2/1 -> Add/2
  Length lower Limb/1 -> Square3/1
  Length upper Limb/1 -> Square2/1
  Square/1 -> Add/1, Add1/1
  Y(t)/1 -> Square1/1
  X(t)/1 -> Square/1, Divide/1

== system gait_testing/Gait Selector/Walk Gait - Bezier Curves/Plane Movement4/Subsystem1 ==
  X(t) : Inport
  Y(t) : Inport  Port=2
  Add : Sum  Inputs=+--+
  Add1 : Sum
  Add2 : Sum
  Asin : Trigonometry  Operator=asin
  Asin1 : Trigonometry  Operator=asin
  Cos : Trigonometry  Operator=acos
  Divide : Product  Inputs=*/
  Divide1 : Product  Inputs=*/
  Gain : Gain  Gain=1/(2*Upper_limbs*Lower_limbs)
  Gain1 : Gain  Gain=Lower_limbs
  Length lower Limb : Constant  Value=Lower_limbs
  Length upper Limb : Constant  Value=Upper_limbs
  Sin : Trigonometry
  Square{,1..3} (4 alike) : Math  Operator=square
  Square Root : Sqrt
  Theta1(X,Y) : Outport
  Theta2(X,Y) : Outport  Port=2
  wires:
  X(t)/1 -> Divide/1, Square/1
  Y(t)/1 -> Square1/1
  Square/1 -> Add1/1, Add/1
  Length upper Limb/1 -> Square2/1
  Length lower Limb/1 -> Square3/1
  Square2/1 -> Add/2
  Square3/1 -> Add/3
  Square1/1 -> Add1/2, Add/4
  Add/1 -> Gain/1
  Gain/1 -> Cos/1
  Cos/1 -> Theta2(X,Y)/1, Sin/1
  Asin/1 -> Add2/1
  Sin/1 -> Gain1/1
  Add1/1 -> Square Root/1
  Gain1/1 -> Divide1/1
  Square Root/1 -> Divide/2, Divide1/2
  Divide1/1 -> Asin1/1
  Asin1/1 -> Add2/2
  Add2/1 -> Theta1(X,Y)/1
  Divide/1 -> Asin/1

== system gait_testing/Gait Selector/Walk Gait - Bezier Curves/Sin-Movement/Subsystem1 ==
  X(t) : Inport
  Y(t) : Inport  Port=2
  Add : Sum  Inputs=+--+
  Add1 : Sum
  Add2 : Sum
  Asin : Trigonometry  Operator=asin
  Asin1 : Trigonometry  Operator=asin
  Cos : Trigonometry  Operator=acos
  Divide : Product  Inputs=*/
  Divide1 : Product  Inputs=*/
  Gain : Gain  Gain=1/(2*Upper_limbs*Lower_limbs)
  Gain1 : Gain  Gain=Lower_limbs
  Length lower Limb : Constant  Value=Lower_limbs
  Length upper Limb : Constant  Value=Upper_limbs
  Sin : Trigonometry
  Square{,1..3} (4 alike) : Math  Operator=square
  Square Root : Sqrt
  Theta1(X,Y) : Outport
  Theta2(X,Y) : Outport  Port=2
  wires:
  Divide/1 -> Asin/1
  Add2/1 -> Theta1(X,Y)/1
  Asin1/1 -> Add2/2
  Divide1/1 -> Asin1/1
  Square Root/1 -> Divide1/2, Divide/2
  Gain1/1 -> Divide1/1
  Add1/1 -> Square Root/1
  Sin/1 -> Gain1/1
  Asin/1 -> Add2/1
  Cos/1 -> Sin/1, Theta2(X,Y)/1
  Gain/1 -> Cos/1
  Add/1 -> Gain/1
  Square1/1 -> Add/4, Add1/2
  Square3/1 -> Add/3
  Square2/1 -> Add/2
  Length lower Limb/1 -> Square3/1
  Length upper Limb/1 -> Square2/1
  Square/1 -> Add/1, Add1/1
  Y(t)/1 -> Square1/1
  X(t)/1 -> Square/1, Divide/1

== system gait_testing/Gait Selector/Walk Gait - Bezier Curves/Stop when change/Triggered Subsystem ==
  t : Inport
  Action Port : ActionPort  InitializeStates=reset  ActionPortLabel=case [ 1 ]:
  MATLAB Function : MATLAB Function  TreatAsAtomicUnit=on
  Change Time : Outport
  wires:
  MATLAB Function/1(activationTime) -> Change Time/1
  t/1 -> MATLAB Function/1(u)

== system gait_testing/Gait Selector/Walk Gait - Bezier Curves/delay and stop when change/Triggered Subsystem ==
  t : Inport
  Action Port : ActionPort  InitializeStates=reset  ActionPortLabel=case [ 1 ]:
  MATLAB Function : MATLAB Function  TreatAsAtomicUnit=on
  Change Time : Outport
  wires:
  MATLAB Function/1(activationTime) -> Change Time/1
  t/1 -> MATLAB Function/1(u)

== system gait_testing/Gait Selector/Walk Gait - Bezier Curves/delay and stop when change1/Triggered Subsystem ==
  t : Inport
  Action Port : ActionPort  InitializeStates=reset  ActionPortLabel=case [ 1 ]:
  MATLAB Function : MATLAB Function  TreatAsAtomicUnit=on
  Change Time : Outport
  wires:
  MATLAB Function/1(activationTime) -> Change Time/1
  t/1 -> MATLAB Function/1(u)

== system gait_testing/Gait Selector/Walk Gait - Bezier Curves/delay and stop when change2/Triggered Subsystem ==
  t : Inport
  Action Port : ActionPort  InitializeStates=reset  ActionPortLabel=case [ 1 ]:
  MATLAB Function : MATLAB Function  TreatAsAtomicUnit=on
  Change Time : Outport
  wires:
  t/1 -> MATLAB Function/1(u)
  MATLAB Function/1(activationTime) -> Change Time/1

== system gait_testing/Gait Selector/Walk Gait - Drive Function/left Back Hip gait/If Action Subsystem ==
  In1 : Inport
  tdur : Inport  Port=2
  Add : Sum  Inputs=+-
  Constant : Constant  Value=1.5 * pi
  Divide : Product  Inputs=*/
  Gain1 : Gain  Gain=2/3
  Gain4 : Gain  Gain=2*pi
  Sin : Trigonometry
  Out1 : Outport
  wires:
  In1/1 -> Gain4/1
  Constant/1 -> Add/2
  Add/1 -> Gain1/1
  Gain1/1 -> Sin/1
  Sin/1 -> Out1/1
  Gain4/1 -> Divide/1
  tdur/1 -> Divide/2
  Divide/1 -> Add/1

== system gait_testing/Gait Selector/Walk Gait - Drive Function/left Back Hip gait/If Action Subsystem1 ==
  In1 : Inport
  tdur : Inport  Port=2
  Add : Sum  Inputs=+-
  Constant : Constant  Value=1.0 * pi
  Divide : Product  Inputs=*/
  Gain1 : Gain  Gain=2
  Gain4 : Gain  Gain=2*pi
  Sin : Trigonometry
  Out1 : Outport
  wires:
  Sin/1 -> Out1/1
  In1/1 -> Gain4/1
  Add/1 -> Gain1/1
  Constant/1 -> Add/2
  Gain1/1 -> Sin/1
  Gain4/1 -> Divide/1
  Divide/1 -> Add/1
  tdur/1 -> Divide/2

== system gait_testing/Gait Selector/Walk Gait - Drive Function/left Back Hip gait/If Action Subsystem2 ==
  In1 : Inport
  tdur : Inport  Port=2
  Add : Sum  Inputs=+-
  Constant : Constant  Value=1.25 * pi
  Divide : Product  Inputs=*/
  Gain1 : Gain  Gain=2/3
  Gain4 : Gain  Gain=2*pi
  Sin : Trigonometry  Operator=cos
  Out1 : Outport
  wires:
  Sin/1 -> Out1/1
  In1/1 -> Gain4/1
  Add/1 -> Gain1/1
  Constant/1 -> Add/2
  Gain1/1 -> Sin/1
  Gain4/1 -> Divide/1
  Divide/1 -> Add/1
  tdur/1 -> Divide/2

== system gait_testing/Gait Selector/Walk Gait - Drive Function/left Back Knee gait/If Action Subsystem4 ==
  In1 : Inport
  tdur : Inport  Port=2
  Add : Sum  Inputs=+-
  Constant : Constant  Value=0.75 * pi
  Divide : Product  Inputs=*/
  Gain1 : Gain  Gain=2
  Gain4 : Gain  Gain=2*pi
  Sin : Trigonometry
  Out1 : Outport
  wires:
  Sin/1 -> Out1/1
  In1/1 -> Gain4/1
  Add/1 -> Gain1/1
  Constant/1 -> Add/2
  Gain1/1 -> Sin/1
  Divide/1 -> Add/1
  Gain4/1 -> Divide/1
  tdur/1 -> Divide/2

== system gait_testing/Gait Selector/Walk Gait - Drive Function/left Fornt Knee gait/If Action Subsystem4 ==
  In1 : Inport
  tdur : Inport  Port=2
  Add : Sum  Inputs=+-
  Constant : Constant  Value=0.75 * pi
  Divide : Product  Inputs=*/
  Gain1 : Gain  Gain=2
  Gain4 : Gain  Gain=2*pi
  Sin : Trigonometry
  Out1 : Outport
  wires:
  Sin/1 -> Out1/1
  In1/1 -> Gain4/1
  Add/1 -> Gain1/1
  Constant/1 -> Add/2
  Gain1/1 -> Sin/1
  Divide/1 -> Add/1
  Gain4/1 -> Divide/1
  tdur/1 -> Divide/2

== system gait_testing/Gait Selector/Walk Gait - Drive Function/left Front Hip gait/If Action Subsystem ==
  In1 : Inport
  tdur : Inport  Port=2
  Add : Sum  Inputs=+-
  Constant : Constant  Value=1.5 * pi
  Divide : Product  Inputs=*/
  Gain1 : Gain  Gain=2/3
  Gain4 : Gain  Gain=2*pi
  Sin : Trigonometry
  Out1 : Outport
  wires:
  In1/1 -> Gain4/1
  Constant/1 -> Add/2
  Add/1 -> Gain1/1
  Gain1/1 -> Sin/1
  Sin/1 -> Out1/1
  Gain4/1 -> Divide/1
  tdur/1 -> Divide/2
  Divide/1 -> Add/1

== system gait_testing/Gait Selector/Walk Gait - Drive Function/left Front Hip gait/If Action Subsystem1 ==
  In1 : Inport
  tdur : Inport  Port=2
  Add : Sum  Inputs=+-
  Constant : Constant  Value=1.0 * pi
  Divide : Product  Inputs=*/
  Gain1 : Gain  Gain=2
  Gain4 : Gain  Gain=2*pi
  Sin : Trigonometry
  Out1 : Outport
  wires:
  Sin/1 -> Out1/1
  In1/1 -> Gain4/1
  Add/1 -> Gain1/1
  Constant/1 -> Add/2
  Gain1/1 -> Sin/1
  Gain4/1 -> Divide/1
  Divide/1 -> Add/1
  tdur/1 -> Divide/2

== system gait_testing/Gait Selector/Walk Gait - Drive Function/left Front Hip gait/If Action Subsystem2 ==
  In1 : Inport
  tdur : Inport  Port=2
  Add : Sum  Inputs=+-
  Constant : Constant  Value=1.25 * pi
  Divide : Product  Inputs=*/
  Gain1 : Gain  Gain=2/3
  Gain4 : Gain  Gain=2*pi
  Sin : Trigonometry  Operator=cos
  Out1 : Outport
  wires:
  Sin/1 -> Out1/1
  In1/1 -> Gain4/1
  Add/1 -> Gain1/1
  Constant/1 -> Add/2
  Gain1/1 -> Sin/1
  Gain4/1 -> Divide/1
  Divide/1 -> Add/1
  tdur/1 -> Divide/2

== system gait_testing/Gait Selector/Walk Gait - Drive Function/right Back Hip gait/If Action Subsystem ==
  In1 : Inport
  tdur : Inport  Port=2
  Add : Sum  Inputs=+-
  Constant : Constant  Value=1.5 * pi
  Divide : Product  Inputs=*/
  Gain1 : Gain  Gain=2/3
  Gain4 : Gain  Gain=2*pi
  Sin : Trigonometry
  Out1 : Outport
  wires:
  In1/1 -> Gain4/1
  Constant/1 -> Add/2
  Add/1 -> Gain1/1
  Gain1/1 -> Sin/1
  Sin/1 -> Out1/1
  Gain4/1 -> Divide/1
  tdur/1 -> Divide/2
  Divide/1 -> Add/1

== system gait_testing/Gait Selector/Walk Gait - Drive Function/right Back Hip gait/If Action Subsystem1 ==
  In1 : Inport
  tdur : Inport  Port=2
  Add : Sum  Inputs=+-
  Constant : Constant  Value=1.0 * pi
  Divide : Product  Inputs=*/
  Gain1 : Gain  Gain=2
  Gain4 : Gain  Gain=2*pi
  Sin : Trigonometry
  Out1 : Outport
  wires:
  Sin/1 -> Out1/1
  In1/1 -> Gain4/1
  Add/1 -> Gain1/1
  Constant/1 -> Add/2
  Gain1/1 -> Sin/1
  Gain4/1 -> Divide/1
  Divide/1 -> Add/1
  tdur/1 -> Divide/2

== system gait_testing/Gait Selector/Walk Gait - Drive Function/right Back Hip gait/If Action Subsystem2 ==
  In1 : Inport
  tdur : Inport  Port=2
  Add : Sum  Inputs=+-
  Constant : Constant  Value=1.25 * pi
  Divide : Product  Inputs=*/
  Gain1 : Gain  Gain=2/3
  Gain4 : Gain  Gain=2*pi
  Sin : Trigonometry  Operator=cos
  Out1 : Outport
  wires:
  Sin/1 -> Out1/1
  In1/1 -> Gain4/1
  Add/1 -> Gain1/1
  Constant/1 -> Add/2
  Gain1/1 -> Sin/1
  Gain4/1 -> Divide/1
  Divide/1 -> Add/1
  tdur/1 -> Divide/2

== system gait_testing/Gait Selector/Walk Gait - Drive Function/right Back Knee gait/If Action Subsystem4 ==
  In1 : Inport
  tdur : Inport  Port=2
  Add : Sum  Inputs=+-
  Constant : Constant  Value=0.75 * pi
  Divide : Product  Inputs=*/
  Gain1 : Gain  Gain=2
  Gain4 : Gain  Gain=2*pi
  Sin : Trigonometry
  Out1 : Outport
  wires:
  Sin/1 -> Out1/1
  In1/1 -> Gain4/1
  Add/1 -> Gain1/1
  Constant/1 -> Add/2
  Gain1/1 -> Sin/1
  Divide/1 -> Add/1
  Gain4/1 -> Divide/1
  tdur/1 -> Divide/2

== system gait_testing/Gait Selector/Walk Gait - Drive Function/right Front Hip gait/If Action Subsystem ==
  In1 : Inport
  tdur : Inport  Port=2
  Add : Sum  Inputs=+-
  Constant : Constant  Value=1.5 * pi
  Divide : Product  Inputs=*/
  Gain1 : Gain  Gain=2/3
  Gain4 : Gain  Gain=2*pi
  Sin : Trigonometry
  Out1 : Outport
  wires:
  In1/1 -> Gain4/1
  Constant/1 -> Add/2
  Add/1 -> Gain1/1
  Gain1/1 -> Sin/1
  Sin/1 -> Out1/1
  Gain4/1 -> Divide/1
  tdur/1 -> Divide/2
  Divide/1 -> Add/1

== system gait_testing/Gait Selector/Walk Gait - Drive Function/right Front Hip gait/If Action Subsystem1 ==
  In1 : Inport
  tdur : Inport  Port=2
  Add : Sum  Inputs=+-
  Constant : Constant  Value=1.0 * pi
  Divide : Product  Inputs=*/
  Gain1 : Gain  Gain=2
  Gain4 : Gain  Gain=2*pi
  Sin : Trigonometry
  Out1 : Outport
  wires:
  Sin/1 -> Out1/1
  In1/1 -> Gain4/1
  Add/1 -> Gain1/1
  Constant/1 -> Add/2
  Gain1/1 -> Sin/1
  Gain4/1 -> Divide/1
  Divide/1 -> Add/1
  tdur/1 -> Divide/2

== system gait_testing/Gait Selector/Walk Gait - Drive Function/right Front Hip gait/If Action Subsystem2 ==
  In1 : Inport
  tdur : Inport  Port=2
  Add : Sum  Inputs=+-
  Constant : Constant  Value=1.25 * pi
  Divide : Product  Inputs=*/
  Gain1 : Gain  Gain=2/3
  Gain4 : Gain  Gain=2*pi
  Sin : Trigonometry  Operator=cos
  Out1 : Outport
  wires:
  Sin/1 -> Out1/1
  In1/1 -> Gain4/1
  Add/1 -> Gain1/1
  Constant/1 -> Add/2
  Gain1/1 -> Sin/1
  Gain4/1 -> Divide/1
  Divide/1 -> Add/1
  tdur/1 -> Divide/2

== system gait_testing/Gait Selector/Walk Gait - Drive Function/right Front Knee gait/If Action Subsystem4 ==
  In1 : Inport
  tdur : Inport  Port=2
  Add : Sum  Inputs=+-
  Constant : Constant  Value=0.75 * pi
  Divide : Product  Inputs=*/
  Gain1 : Gain  Gain=2
  Gain4 : Gain  Gain=2*pi
  Sin : Trigonometry
  Out1 : Outport
  wires:
  Sin/1 -> Out1/1
  In1/1 -> Gain4/1
  Add/1 -> Gain1/1
  Constant/1 -> Add/2
  Gain1/1 -> Sin/1
  Divide/1 -> Add/1
  Gain4/1 -> Divide/1
  tdur/1 -> Divide/2
